simulink model "RadarSimulinkProjectRev008"  (R2024a)
settings: Solver=VariableStepAuto  StartTime=0.0  StopTime=0.0125  RelTol=1e-3
values from neighbouring files (symbols this model uses):
  AngleTime = SweepTime/10    (= 10000)    [InitializationOfVariablesRev000.m]    (also in InitializationOfVariablesRev001.m; InitializationOfVariablesRev002.m = 2000; InitializationOfVariablesRev003.m = 20000; InitializationOfVariablesRev004.m = 2097152)
  ASR_LUT = Rsamp    [InitializationOfVariablesRev003.m]    (also in InitializationOfVariablesRev004.m = round((R*2*SystemFs)/c); InitializationOfVariablesRev005.m = round((R*2*SystemFs)/c))
  Btn_Debounce = 20000    [InitializationOfVariablesRev003.m]    (also in InitializationOfVariablesRev004.m; InitializationOfVariablesRev005.m)
  ChirpNc = 128    [InitializationOfVariablesRev004.m]    (also in InitializationOfVariablesRev005.m)
  ChirpSizeLength = length(FCW)    [InitializationOfVariablesRev004.m]    (also in InitializationOfVariablesRev005.m = 16384)
  DeciFactor = 8    [InitializationOfVariablesRev005.m]
  FCW = [FCW_p1, FCW_p2]    [InitializationOfVariablesRev002.m]    (also in InitializationOfVariablesRev003.m; InitializationOfVariablesRev004.m = interp1(1:length(FCW_base), FCW_base,      linspace(1, lengt; InitializationOfVariablesRev005.m = f / SystemFs)
  filt1divide = sum(h1_int)    [InitializationOfVariablesRev004.m]
  RXFFTLength = 4096    [InitializationOfVariablesRev003.m]    (also in InitializationOfVariablesRev004.m = 1024; InitializationOfVariablesRev005.m = 2048)
  SweepTime = 100000    [InitializationOfVariablesRev000.m]    (also in InitializationOfVariablesRev001.m; InitializationOfVariablesRev002.m = 20000; InitializationOfVariablesRev003.m = 200000; InitializationOfVariablesRev004.m = 23068672)
undefined symbols (not defined in the file or in its folder): SignalGenerationForAnalysis, Subsystem, xc7a200tfbg676
libraries: hdlBasic x362, hdlDSPIP x15, hdlUtilities x11, vmcUtilities x1
(part 3 of 4)

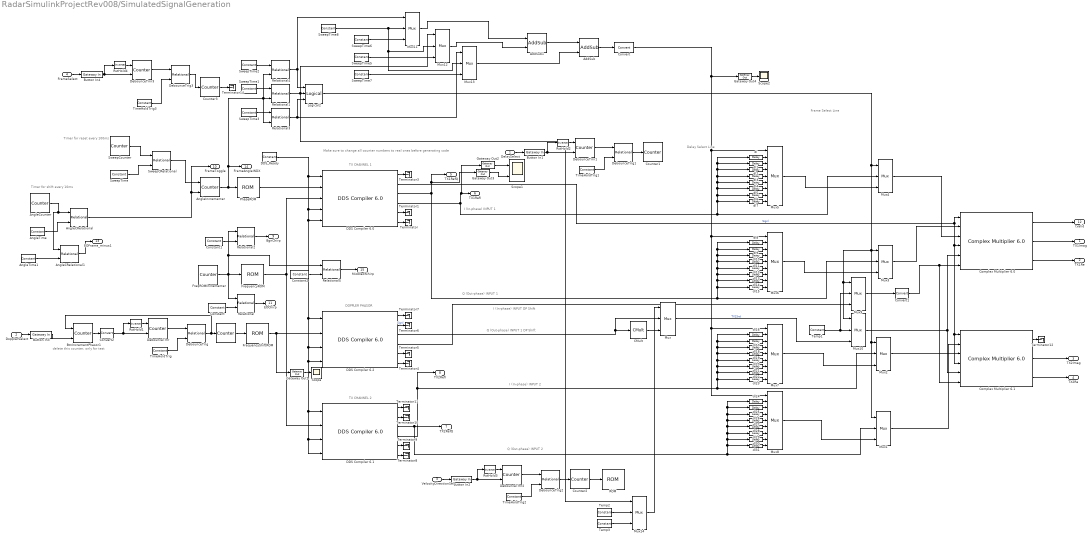
== system RadarSimulinkProjectRev008/SimulatedSignalGeneration ==
  note: delete this counter, only for test
  note: TX CHANNEL 1
  note: Frame Select Line
  note: Make sure to change all counter numbers to real ones before generating code
  note: Timer for shift every 10ms
  note: Timer for reset every 100ms
  note: I (In-phase) INPUT 1
  note: Q (Out-phase) INPUT 1
  note: Q (Out-phase) INPUT 2
  note: Q (Out-phase) INPUT 1 DP Shift
  note: I (In-phase) INPUT DP Shift
  note: I (In-phase) INPUT 2
  note: Delay Select Line
  note: TX CHANNEL 2
  note: DOPPLER PHASOR
  DelaySelect : Inport
  DopplerSelect : Inport  Port=2
  VelocityDirectionSel : Inport  Port=3
  FrameSelect : Inport  Port=4
  " " : hdlBasic/Counter  cnt_type=Count limited  cnt_to=8  operation=Up  start_count=6  cnt_by_val=1  arith_type=Unsigned  n_bits=4  bin_pt=0  load_pin=off  rst=off  en=on  explicit_period=Explicit  period=P1  use_behavioral_HDL=off  implementation=Fabric  XmcBlockStatus=1  maskContainerNames=group1  block_type=counter  block_config=sysgen:Counter_config  block_width=531  block_height=1023
  AddSub : hdlBasic/AddSub  mode=Addition  use_carryin=off  use_carryout=off  en=off  latency=0  precision=Full  arith_type=Unsigned  n_bits=16  bin_pt=14  quantization=Truncate  overflow=Wrap  use_behavioral_HDL=off  hw_selection=Fabric  pipelined=off  XmcBlockStatus=1  maskContainerNames=tabcontainer1  block_type=addsub  block_config=sysgen:Addsub_config
  AddSub1 : hdlBasic/AddSub  mode=Addition  use_carryin=off  use_carryout=off  en=off  latency=0  precision=Full  arith_type=Unsigned  n_bits=16  bin_pt=14  quantization=Truncate  overflow=Wrap  use_behavioral_HDL=off  hw_selection=Fabric  pipelined=off  XmcBlockStatus=1  maskContainerNames=tabcontainer1  block_type=addsub  block_config=sysgen:Addsub_config
  AngleCRelational : hdlBasic/Relational  mode=a=b  op_type=Bool  en=off  latency=0  XmcBlockStatus=1  maskContainerNames=tabcontainer1  block_type=relational  block_config=sysgen:Relational_config
  AngleCRelational1 : hdlBasic/Relational  mode=a=b  op_type=Bool  en=off  latency=0  XmcBlockStatus=1  maskContainerNames=tabcontainer1  block_type=relational  block_config=sysgen:Relational_config
  AngleCounter : hdlBasic/Counter  cnt_type=Count limited  cnt_to=AngleTime-1  operation=Up  start_count=0  cnt_by_val=1  arith_type=Unsigned  n_bits=32  bin_pt=0  load_pin=off  rst=off  en=off  explicit_period=Explicit  period=P1  use_behavioral_HDL=off  implementation=Fabric  XmcBlockStatus=1  maskContainerNames=group1  block_type=counter  block_config=sysgen:Counter_config  block_width=531  block_height=1023
  AngleIncrementer : hdlBasic/Counter  cnt_type=Count limited  cnt_to=10  operation=Up  start_count=0  cnt_by_val=1  arith_type=Unsigned  n_bits=4  bin_pt=0  load_pin=off  rst=on  en=on  explicit_period=Explicit  period=P1  use_behavioral_HDL=off  implementation=Fabric  XmcBlockStatus=1  maskContainerNames=group1  block_type=counter  block_config=sysgen:Counter_config  block_width=531  block_height=1023
  AngleTime : hdlBasic/Constant  const=AngleTime-1  gui_display_data_type=Fixed-point  arith_type=Unsigned  n_bits=24  bin_pt=0  preci_type=Single  exp_width=8  frac_width=24  explicit_period=off  period=1  XmcBlockStatus=1  maskContainerNames=tabcontainer1  block_type=constant  block_config=sysgen:Constant_config
  AngleTime1 : hdlBasic/Constant  const=AngleTime-2  gui_display_data_type=Fixed-point  arith_type=Unsigned  n_bits=24  bin_pt=0  preci_type=Single  exp_width=8  frac_width=24  explicit_period=off  period=1  XmcBlockStatus=1  maskContainerNames=tabcontainer1  block_type=constant  block_config=sysgen:Constant_config
  BtnIncrementPhasor1 : hdlBasic/Counter  cnt_type=Count limited  cnt_to=1  operation=Up  start_count=0  cnt_by_val=1  arith_type=Unsigned  n_bits=1  bin_pt=0  load_pin=off  rst=on  en=on  explicit_period=Explicit  period=P1  use_behavioral_HDL=off  implementation=Fabric  XmcBlockStatus=1  maskContainerNames=group1  block_type=counter  block_config=sysgen:Counter_config  block_width=531  block_height=1023
  Button In{1..4} (4 alike) : hdlBasic/Gateway In  gui_display_data_type=Boolean  arith_type=Boolean  n_bits=16  bin_pt=14  preci_type=Single  exp_width=8  frac_width=24  rows=1  columns=1  quantization="Round  (unbiased: +/- Inf)"  overflow=Saturate  period=P1  UseAsADC=off  ADCChannel='1'  interface=None  automatic_assignment=on  address_offset=hex2dec('00')  intf_name=''  intf_description=''  default_value=0  timing_constraint=None  locs_specified=off  LOCs={}  io_standard={}  inherit_from_input=off  hdl_port=on  XmcBlockStatus=1  maskContainerNames=group4  block_type=gatewayin  block_config=sysgen:gateway_in_config  block_width_w=590  block_height_w=620  block_width=640  block_height=850
  CMult : hdlBasic/CMult  const=-1  gui_display_data_type=Fixed-point  const_n_bits=1  const_bin_pt=0  float_type=Single  exp_bits=8  fraction_bits=24  en=off  latency=0  precision=Full  arith_type="Signed  (2's comp)"  n_bits=16  bin_pt=14  quantization=Truncate  overflow=Wrap  use_behavioral_HDL=off  mem_type=Distributed RAM  pipeline=off  XmcBlockStatus=1  maskContainerNames=tabcontainer1  block_type=cmult  block_config=sysgen:CMult_config
      settings: infoedit=[]
  Complex Multiplier 6.0 : hdlDSPIP/Complex Multiplier 6.0   datatype=integer  hasatlast=off  hasatuser=off  atuserwidth=1  hasbtlast=off  hasbtuser=off  btuserwidth=1  multtype=Use_Mults  optimizegoal=Resources  flowcontrol=NonBlocking  outputwidth=34  roundmode=Truncate  hasctrltlast=off  hasctrltuser=off  ctrltuserwidth=1  outtlastbehv=Null  latencyconfig=Manual  minimumlatency=50  aclken=off  aresetn=off  trim_axipin_name=on  simulation_type=hybrid_sim  simulation_model=sysgen:cmpy_v6_0  data_path_portlist={ 's_axis_a_tdata_real', 's_axis_a_tdata_imag', 's_axis_b_tdata_real', 's_axis_b_tdata_imag', 's_axis_ctrl_tdata_rounding_bit', 'm_axis_dout_tdata_real', 'm_axis_dout_tdata_imag' }  aportwidth=63  bportwidth=63  ip_name=Complex Multiplier  ip_version=6.0  dsptool_ready=true  ipcore_usecache=true  ipcore_useipmodelcache=true  ipcore_verbose=false  ipcore_latency_parameter='minimumlatency'  wrapper_available=true  port_translation_map={ 'aclken' => 'en', 'aresetn' => 'rst'}  XmcBlockStatus=1  maskContainerNames=tabcontainer1  block_type=cmpy_v6_0  block_config=sysgen:rodinimport_config
  Complex Multiplier 6.1 : hdlDSPIP/Complex Multiplier 6.0   datatype=integer  hasatlast=off  hasatuser=off  atuserwidth=1  hasbtlast=off  hasbtuser=off  btuserwidth=1  multtype=Use_Mults  optimizegoal=Resources  flowcontrol=NonBlocking  outputwidth=34  roundmode=Truncate  hasctrltlast=off  hasctrltuser=off  ctrltuserwidth=1  outtlastbehv=Null  latencyconfig=Manual  minimumlatency=50  aclken=off  aresetn=off  trim_axipin_name=on  simulation_type=hybrid_sim  simulation_model=sysgen:cmpy_v6_0  data_path_portlist={ 's_axis_a_tdata_real', 's_axis_a_tdata_imag', 's_axis_b_tdata_real', 's_axis_b_tdata_imag', 's_axis_ctrl_tdata_rounding_bit', 'm_axis_dout_tdata_real', 'm_axis_dout_tdata_imag' }  aportwidth=63  bportwidth=63  ip_name=Complex Multiplier  ip_version=6.0  dsptool_ready=true  ipcore_usecache=true  ipcore_useipmodelcache=true  ipcore_verbose=false  ipcore_latency_parameter='minimumlatency'  wrapper_available=true  port_translation_map={ 'aclken' => 'en', 'aresetn' => 'rst'}  XmcBlockStatus=1  maskContainerNames=tabcontainer1  block_type=cmpy_v6_0  block_config=sysgen:rodinimport_config
  Constant : hdlBasic/Constant  const=length(FCW)-1  gui_display_data_type=Fixed-point  arith_type=Unsigned  n_bits=14  bin_pt=0  preci_type=Single  exp_width=8  frac_width=24  explicit_period=off  period=1  XmcBlockStatus=1  maskContainerNames=tabcontainer1  block_type=constant  block_config=sysgen:Constant_config
  Constant1 : hdlBasic/Constant  const=0  gui_display_data_type=Fixed-point  arith_type=Unsigned  n_bits=12  bin_pt=0  preci_type=Single  exp_width=8  frac_width=24  explicit_period=off  period=1  XmcBlockStatus=1  maskContainerNames=tabcontainer1  block_type=constant  block_config=sysgen:Constant_config
  Constant2 : hdlBasic/Constant  const=(length(FCW)/2)-1  gui_display_data_type=Fixed-point  arith_type=Unsigned  n_bits=13  bin_pt=0  preci_type=Single  exp_width=8  frac_width=24  explicit_period=off  period=1  XmcBlockStatus=1  maskContainerNames=tabcontainer1  block_type=constant  block_config=sysgen:Constant_config
  Convert : hdlBasic/Convert  gui_display_data_type=Fixed-point  arith_type=Unsigned  n_bits=3  bin_pt=0  float_type=Single  exp_bits=8  fraction_bits=24  quantization=Truncate  overflow=Wrap  en=off  latency=0  pipeline=off  XmcBlockStatus=1  maskContainerNames=group2  block_type=convert  block_config=sysgen:Convert_config  block_width=595  block_height=885
  Convert1 : hdlBasic/Convert  gui_display_data_type=Fixed-point  arith_type=Signed (2's comp)  n_bits=17  bin_pt=15  float_type=Single  exp_bits=8  fraction_bits=24  quantization=Truncate  overflow=Saturate  en=off  latency=0  pipeline=off  XmcBlockStatus=1  maskContainerNames=group2  block_type=convert  block_config=sysgen:Convert_config  block_width=595  block_height=885
  Convert2 : hdlBasic/Convert  gui_display_data_type=Boolean  arith_type=Boolean  n_bits=17  bin_pt=15  float_type=Single  exp_bits=8  fraction_bits=24  quantization=Truncate  overflow=Wrap  en=off  latency=0  pipeline=off  XmcBlockStatus=1  maskContainerNames=group2  block_type=convert  block_config=sysgen:Convert_config  block_width=595  block_height=885
  Counter1 : hdlBasic/Counter  cnt_type=Count limited  cnt_to=7  operation=Up  start_count=0  cnt_by_val=1  arith_type=Unsigned  n_bits=3  bin_pt=0  load_pin=off  rst=off  en=on  explicit_period=Explicit  period=P1  use_behavioral_HDL=off  implementation=Fabric  XmcBlockStatus=1  maskContainerNames=group1  block_type=counter  block_config=sysgen:Counter_config  block_width=531  block_height=1023
  Counter2 : hdlBasic/Counter  cnt_type=Count limited  cnt_to=1  operation=Up  start_count=0  cnt_by_val=1  arith_type=Unsigned  n_bits=1  bin_pt=0  load_pin=off  rst=off  en=on  explicit_period=Explicit  period=P1  use_behavioral_HDL=off  implementation=Fabric  XmcBlockStatus=1  maskContainerNames=group1  block_type=counter  block_config=sysgen:Counter_config  block_width=531  block_height=1023
  Counter3 : hdlBasic/Counter  cnt_type=Count limited  cnt_to=10  operation=Up  start_count=0  cnt_by_val=1  arith_type=Unsigned  n_bits=4  bin_pt=0  load_pin=off  rst=off  en=on  explicit_period=Explicit  period=P1  use_behavioral_HDL=off  implementation=Fabric  XmcBlockStatus=1  maskContainerNames=group1  block_type=counter  block_config=sysgen:Counter_config  block_width=531  block_height=1023
  DDS Compiler 6.0 : hdlDSPIP/DDS Compiler 6.0   partspresent=Phase_Generator_and_SIN_COS_LUT  dds_clock_rate=200  channels=1  mode_of_operation=Standard  output_type=Integer  modulus=9  parameter_entry=Hardware_Parameters  spurious_free_dynamic_range=45  frequency_resolution=0.4  noise_shaping=None  phase_width=24  output_width=16  output_selection=Sine_and_Cosine  negative_sine=off  negative_cosine=off  amplitude_mode=Full_Range  memory_type=Auto  optimization_goal=Auto  dsp48_use=Minimal  resync=off  latency_configuration=Auto  latency=1  has_phase_out=on  has_aclken=off  has_aresetn=off  explicit_period=on  period=P1  data_has_tlast=Not_Required  has_tready=on  s_phase_has_tuser=Not_Required  m_data_has_tuser=Not_Required  m_phase_has_tuser=Not_Required  s_phase_tuser_width=1  output_form=Twos_Complement  s_config_sync_mode=On_Vector  phase_increment=Streaming  output_frequency1=0  output_frequency2=0  output_frequency3=0  output_frequency4=0  output_frequency5=0  output_frequency6=0  output_frequency7=0  output_frequency8=0  output_frequency9=0  output_frequency10=0  output_frequency11=0  output_frequency12=0  output_frequency13=0  output_frequency14=0  output_frequency15=0  output_frequency16=0  pinc1='0'  pinc2='0'  pinc3='0'  pinc4='0'  pinc5='0'  pinc6='0'  pinc7='0'  pinc8='0'  pinc9='0'  pinc10='0'  pinc11='0'  pinc12='0'  pinc13='0'  pinc14='0'  pinc15='0'  pinc16='0'  phase_offset=Streaming  phase_offset_angles1=0  phase_offset_angles2=0  phase_offset_angles3=0  phase_offset_angles4=0  phase_offset_angles5=0  phase_offset_angles6=0  phase_offset_angles7=0  phase_offset_angles8=0  phase_offset_angles9=0  phase_offset_angles10=0  phase_offset_angles11=0  phase_offset_angles12=0  phase_offset_angles13=0  phase_offset_angles14=0  phase_offset_angles15=0  phase_offset_angles16=0  poff1='0'  poff2='0'  poff3='0'  poff4='0'  poff5='0'  poff6='0'  poff7='0'  poff8='0'  poff9='0'  poff10='0'  poff11='0'  poff12='0'  poff13='0'  poff14='0'  poff15='0'  poff16='0'  trim_axipin_name=on  simulation_type=hybrid_sim  simulation_model=sysgen:xddsv6_0_cmodel  data_path_portlist={ 's_axis_config_tdata_poff', 's_axis_config_tdata_chan0_poff', 's_axis_config_tdata_pinc', 's_axis_config_tdata_chan0_pinc', 's_axis_phase_tdata_resync', 's_axis_phase_tdata_chan0_resync', 's_axis_phase_tdata_poff', 's_axis_phase_tdata_chan0_poff', 's_axis_phase_tdata_pinc', 's_axis_phase_tdata_chan0_pinc', 's_axis_phase_tdata_phase_in', 'm_axis_data_tdata_sine', 'm_axis_data_tdata_chan0_sine', 'm_axis_data_tdata_cosine', 'm_axis_data_tdata_chan0_cosine', 'm_axis_phase_tdata_phase_out', 'm_axis_phase_tdata_chan0_phase_out'}  por_mode=false  gui_behaviour=Sysgen  ip_name=DDS Compiler  ip_version=6.0  dsptool_ready=true  wrapper_available=true  port_translation_map={ 'aclken' => 'en', 'aresetn' => 'rst' }  ipcore_usecache=true  ipcore_useipmodelcache=true  ipcore_xco_need_fpga_part=true  ipcore_fpga_part=[]  ipcore_verbose=false  XmcBlockStatus=1  maskContainerNames=tabcontainer1  block_type=dds_compiler_v6_0  block_config=sysgen:rodinimport_config  block_width=760
  DDS Compiler 6.1 : hdlDSPIP/DDS Compiler 6.0   partspresent=Phase_Generator_and_SIN_COS_LUT  dds_clock_rate=200  channels=1  mode_of_operation=Standard  output_type=Integer  modulus=9  parameter_entry=Hardware_Parameters  spurious_free_dynamic_range=45  frequency_resolution=0.4  noise_shaping=None  phase_width=24  output_width=16  output_selection=Sine_and_Cosine  negative_sine=off  negative_cosine=off  amplitude_mode=Full_Range  memory_type=Auto  optimization_goal=Auto  dsp48_use=Minimal  resync=off  latency_configuration=Auto  latency=1  has_phase_out=on  has_aclken=off  has_aresetn=off  explicit_period=on  period=P1  data_has_tlast=Not_Required  has_tready=on  s_phase_has_tuser=Not_Required  m_data_has_tuser=Not_Required  m_phase_has_tuser=Not_Required  s_phase_tuser_width=1  output_form=Twos_Complement  s_config_sync_mode=On_Vector  phase_increment=Streaming  output_frequency1=0  output_frequency2=0  output_frequency3=0  output_frequency4=0  output_frequency5=0  output_frequency6=0  output_frequency7=0  output_frequency8=0  output_frequency9=0  output_frequency10=0  output_frequency11=0  output_frequency12=0  output_frequency13=0  output_frequency14=0  output_frequency15=0  output_frequency16=0  pinc1='0'  pinc2='0'  pinc3='0'  pinc4='0'  pinc5='0'  pinc6='0'  pinc7='0'  pinc8='0'  pinc9='0'  pinc10='0'  pinc11='0'  pinc12='0'  pinc13='0'  pinc14='0'  pinc15='0'  pinc16='0'  phase_offset=Fixed  phase_offset_angles1=0  phase_offset_angles2=0  phase_offset_angles3=0  phase_offset_angles4=0  phase_offset_angles5=0  phase_offset_angles6=0  phase_offset_angles7=0  phase_offset_angles8=0  phase_offset_angles9=0  phase_offset_angles10=0  phase_offset_angles11=0  phase_offset_angles12=0  phase_offset_angles13=0  phase_offset_angles14=0  phase_offset_angles15=0  phase_offset_angles16=0  poff1='0'  poff2='0'  poff3='0'  poff4='0'  poff5='0'  poff6='0'  poff7='0'  poff8='0'  poff9='0'  poff10='0'  poff11='0'  poff12='0'  poff13='0'  poff14='0'  poff15='0'  poff16='0'  trim_axipin_name=on  simulation_type=hybrid_sim  simulation_model=sysgen:xddsv6_0_cmodel  data_path_portlist={ 's_axis_config_tdata_poff', 's_axis_config_tdata_chan0_poff', 's_axis_config_tdata_pinc', 's_axis_config_tdata_chan0_pinc', 's_axis_phase_tdata_resync', 's_axis_phase_tdata_chan0_resync', 's_axis_phase_tdata_poff', 's_axis_phase_tdata_chan0_poff', 's_axis_phase_tdata_pinc', 's_axis_phase_tdata_chan0_pinc', 's_axis_phase_tdata_phase_in', 'm_axis_data_tdata_sine', 'm_axis_data_tdata_chan0_sine', 'm_axis_data_tdata_cosine', 'm_axis_data_tdata_chan0_cosine', 'm_axis_phase_tdata_phase_out', 'm_axis_phase_tdata_chan0_phase_out'}  por_mode=false  gui_behaviour=Sysgen  ip_name=DDS Compiler  ip_version=6.0  dsptool_ready=true  wrapper_available=true  port_translation_map={ 'aclken' => 'en', 'aresetn' => 'rst' }  ipcore_usecache=true  ipcore_useipmodelcache=true  ipcore_xco_need_fpga_part=true  ipcore_fpga_part=[]  ipcore_verbose=false  XmcBlockStatus=1  maskContainerNames=tabcontainer1  block_type=dds_compiler_v6_0  block_config=sysgen:rodinimport_config  block_width=760
  DDS Compiler 6.2 : hdlDSPIP/DDS Compiler 6.0   partspresent=Phase_Generator_and_SIN_COS_LUT  dds_clock_rate=200  channels=1  mode_of_operation=Standard  output_type=Integer  modulus=9  parameter_entry=Hardware_Parameters  spurious_free_dynamic_range=45  frequency_resolution=0.4  noise_shaping=None  phase_width=24  output_width=16  output_selection=Sine_and_Cosine  negative_sine=off  negative_cosine=off  amplitude_mode=Full_Range  memory_type=Auto  optimization_goal=Auto  dsp48_use=Minimal  resync=off  latency_configuration=Auto  latency=1  has_phase_out=on  has_aclken=off  has_aresetn=off  explicit_period=on  period=P1  data_has_tlast=Not_Required  has_tready=on  s_phase_has_tuser=Not_Required  m_data_has_tuser=Not_Required  m_phase_has_tuser=Not_Required  s_phase_tuser_width=1  output_form=Twos_Complement  s_config_sync_mode=On_Vector  phase_increment=Streaming  output_frequency1=0  output_frequency2=0  output_frequency3=0  output_frequency4=0  output_frequency5=0  output_frequency6=0  output_frequency7=0  output_frequency8=0  output_frequency9=0  output_frequency10=0  output_frequency11=0  output_frequency12=0  output_frequency13=0  output_frequency14=0  output_frequency15=0  output_frequency16=0  pinc1='0'  pinc2='0'  pinc3='0'  pinc4='0'  pinc5='0'  pinc6='0'  pinc7='0'  pinc8='0'  pinc9='0'  pinc10='0'  pinc11='0'  pinc12='0'  pinc13='0'  pinc14='0'  pinc15='0'  pinc16='0'  phase_offset=None  phase_offset_angles1=0  phase_offset_angles2=0  phase_offset_angles3=0  phase_offset_angles4=0  phase_offset_angles5=0  phase_offset_angles6=0  phase_offset_angles7=0  phase_offset_angles8=0  phase_offset_angles9=0  phase_offset_angles10=0  phase_offset_angles11=0  phase_offset_angles12=0  phase_offset_angles13=0  phase_offset_angles14=0  phase_offset_angles15=0  phase_offset_angles16=0  poff1='0'  poff2='0'  poff3='0'  poff4='0'  poff5='0'  poff6='0'  poff7='0'  poff8='0'  poff9='0'  poff10='0'  poff11='0'  poff12='0'  poff13='0'  poff14='0'  poff15='0'  poff16='0'  trim_axipin_name=on  simulation_type=hybrid_sim  simulation_model=sysgen:xddsv6_0_cmodel  data_path_portlist={ 's_axis_config_tdata_poff', 's_axis_config_tdata_chan0_poff', 's_axis_config_tdata_pinc', 's_axis_config_tdata_chan0_pinc', 's_axis_phase_tdata_resync', 's_axis_phase_tdata_chan0_resync', 's_axis_phase_tdata_poff', 's_axis_phase_tdata_chan0_poff', 's_axis_phase_tdata_pinc', 's_axis_phase_tdata_chan0_pinc', 's_axis_phase_tdata_phase_in', 'm_axis_data_tdata_sine', 'm_axis_data_tdata_chan0_sine', 'm_axis_data_tdata_cosine', 'm_axis_data_tdata_chan0_cosine', 'm_axis_phase_tdata_phase_out', 'm_axis_phase_tdata_chan0_phase_out'}  por_mode=false  gui_behaviour=Sysgen  ip_name=DDS Compiler  ip_version=6.0  dsptool_ready=true  wrapper_available=true  port_translation_map={ 'aclken' => 'en', 'aresetn' => 'rst' }  ipcore_usecache=true  ipcore_useipmodelcache=true  ipcore_xco_need_fpga_part=true  ipcore_fpga_part=[]  ipcore_verbose=false  XmcBlockStatus=1  maskContainerNames=tabcontainer1  block_type=dds_compiler_v6_0  block_config=sysgen:rodinimport_config  block_width=760
  DDS_Ready : hdlBasic/Constant  const=1  gui_display_data_type=Boolean  arith_type=Boolean  n_bits=24  bin_pt=0  preci_type=Single  exp_width=8  frac_width=24  explicit_period=on  period=P1  XmcBlockStatus=1  maskContainerNames=tabcontainer1  block_type=constant  block_config=sysgen:Constant_config
  DebounceTmr{,1..3} (4 alike) : hdlBasic/Counter  cnt_type=Count limited  cnt_to=Btn_Debounce-1  operation=Up  start_count=0  cnt_by_val=1  arith_type=Unsigned  n_bits=18  bin_pt=0  load_pin=off  rst=on  en=on  explicit_period=Explicit  period=P1  use_behavioral_HDL=off  implementation=Fabric  XmcBlockStatus=1  maskContainerNames=group1  block_type=counter  block_config=sysgen:Counter_config  block_width=531  block_height=1023
  DebounceTrig{,1..3} (4 alike) : hdlBasic/Relational  mode=a=b  op_type=Bool  en=off  latency=1  XmcBlockStatus=1  maskContainerNames=tabcontainer1  block_type=relational  block_config=sysgen:Relational_config
  FreqROMIncrementer : hdlBasic/Counter  cnt_type=Count limited  cnt_to=length(FCW)-1  operation=Up  start_count=0  cnt_by_val=1  arith_type=Unsigned  n_bits=14  bin_pt=0  load_pin=off  rst=off  en=off  explicit_period=Explicit  period=P1  use_behavioral_HDL=off  implementation=Fabric  XmcBlockStatus=1  maskContainerNames=group1  block_type=counter  block_config=sysgen:Counter_config  block_width=531  block_height=1023
  FrequencyROM : hdlBasic/ROM  depth=length(FCW)  initVector=FCW  distributed_mem=Block RAM  rst=off  init_reg=0  en=off  latency=1  gui_display_data_type=Fixed-point  arith_type=Unsigned  n_bits=24  bin_pt=24  preci_type=Double  exp_width=8  frac_width=24  optimize=Area  use_rpm=on  simulation_type=fast_sim  XmcBlockStatus=1  maskContainerNames=tabcontainer1  block_type=sprom  block_config=sysgen:SPROM_config
  FrequencyShiftROM : hdlBasic/ROM  depth=9  initVector=DPShift  distributed_mem=Block RAM  rst=off  init_reg=0  en=off  latency=1  gui_display_data_type=Fixed-point  arith_type=Unsigned  n_bits=24  bin_pt=24  preci_type=Double  exp_width=8  frac_width=24  optimize=Area  use_rpm=on  simulation_type=fast_sim  XmcBlockStatus=1  maskContainerNames=tabcontainer1  block_type=sprom  block_config=sysgen:SPROM_config
  Gateway Out{1..4} (4 alike) : hdlBasic/Gateway Out  inherit_from_input=off  bool_to_boolean=off  hdl_port=on  rows=1  columns=1  UseAsDAC=off  DACChannel='1'  interface=None  automatic_assignment=on  address_offset=hex2dec('00')  intf_name=''  intf_description=''  timing_constraint=None  locs_specified=off  LOCs={}  io_standard={}  XmcBlockStatus=1  maskContainerNames=group4  block_type=gatewayout  block_config=sysgen:gateway_out_config  block_width_w=590  block_height_w=620  block_width=620  block_height=750
  Logical2 : hdlBasic/Logical  logical_function=OR  inputs=3  en=off  latency=0  precision=Full  arith_type=Unsigned  n_bits=16  bin_pt=0  align_bp=on  overflow=[]  quantization=[]  XmcBlockStatus=1  maskContainerNames=tabcontainer1  block_type=logical  block_config=sysgen:Logical_config
  Mux{,1..4,9..14} (11 alike) : hdlBasic/Mux  inputs=2  en=off  latency=0  precision=Full  arith_type=Unsigned  n_bits=16  bin_pt=14  quantization=Truncate  overflow=Wrap  XmcBlockStatus=1  maskContainerNames=tabcontainer1  block_type=mux  block_config=sysgen:Mux_config
  Mux{5..8} (4 alike) : hdlBasic/Mux  inputs=8  en=off  latency=0  precision=Full  arith_type=Unsigned  n_bits=16  bin_pt=14  quantization=Truncate  overflow=Wrap  XmcBlockStatus=1  maskContainerNames=tabcontainer1  block_type=mux  block_config=sysgen:Mux_config
  PhaseROM : hdlBasic/ROM  depth=11  initVector=phi_norm  distributed_mem=Block RAM  rst=off  init_reg=0  en=off  latency=1  gui_display_data_type=Fixed-point  arith_type=Unsigned  n_bits=24  bin_pt=24  preci_type=Double  exp_width=8  frac_width=24  optimize=Area  use_rpm=on  simulation_type=fast_sim  XmcBlockStatus=1  maskContainerNames=tabcontainer1  block_type=sprom  block_config=sysgen:SPROM_config
  ROM : hdlBasic/ROM  depth=2  initVector=[0,1]  distributed_mem=Block RAM  rst=off  init_reg=0  en=off  latency=1  gui_display_data_type=Boolean  arith_type=Boolean  n_bits=16  bin_pt=14  preci_type=Single  exp_width=8  frac_width=24  optimize=Area  use_rpm=on  simulation_type=fast_sim  XmcBlockStatus=1  maskContainerNames=tabcontainer1  block_type=sprom  block_config=sysgen:SPROM_config
  Relational : hdlBasic/Relational  mode=a=b  op_type=Bool  en=off  latency=0  XmcBlockStatus=1  maskContainerNames=tabcontainer1  block_type=relational  block_config=sysgen:Relational_config
  Relational1 : hdlBasic/Relational  mode=a=b  op_type=Bool  en=off  latency=1  XmcBlockStatus=1  maskContainerNames=tabcontainer1  block_type=relational  block_config=sysgen:Relational_config
  Relational2 : hdlBasic/Relational  mode=a=b  op_type=Bool  en=off  latency=0  XmcBlockStatus=1  maskContainerNames=tabcontainer1  block_type=relational  block_config=sysgen:Relational_config
  Relational3 : hdlBasic/Relational  mode=a=b  op_type=Bool  en=off  latency=1  XmcBlockStatus=1  maskContainerNames=tabcontainer1  block_type=relational  block_config=sysgen:Relational_config
  Relational4 : hdlBasic/Relational  mode=a=b  op_type=Bool  en=off  latency=1  XmcBlockStatus=1  maskContainerNames=tabcontainer1  block_type=relational  block_config=sysgen:Relational_config
  Relational5 : hdlBasic/Relational  mode=a=b  op_type=Bool  en=off  latency=0  XmcBlockStatus=1  maskContainerNames=tabcontainer1  block_type=relational  block_config=sysgen:Relational_config
  RstHold{1..4} (4 alike) : hdlBasic/Inverter  en=off  latency=0  XmcBlockStatus=1  maskContainerNames=group2  block_type=inv  block_config=sysgen:Inverter_config
  Scope : Scope
  Scope1 : Scope  NumInputPorts=2
  Scope2 : Scope
  SweepCRelational : hdlBasic/Relational  mode=a=b  op_type=Bool  en=off  latency=0  XmcBlockStatus=1  maskContainerNames=tabcontainer1  block_type=relational  block_config=sysgen:Relational_config
  SweepCounter : hdlBasic/Counter  cnt_type=Count limited  cnt_to=SweepTime-1  operation=Up  start_count=0  cnt_by_val=1  arith_type=Unsigned  n_bits=32  bin_pt=0  load_pin=off  rst=off  en=off  explicit_period=Explicit  period=P1  use_behavioral_HDL=off  implementation=Fabric  XmcBlockStatus=1  maskContainerNames=group1  block_type=counter  block_config=sysgen:Counter_config  block_width=531  block_height=1023
  SweepTime : hdlBasic/Constant  const=SweepTime-1  gui_display_data_type=Fixed-point  arith_type=Unsigned  n_bits=32  bin_pt=0  preci_type=Single  exp_width=8  frac_width=24  explicit_period=off  period=1  XmcBlockStatus=1  maskContainerNames=tabcontainer1  block_type=constant  block_config=sysgen:Constant_config
  SweepTime1 : hdlBasic/Constant  const=5  gui_display_data_type=Fixed-point  arith_type=Unsigned  n_bits=4  bin_pt=0  preci_type=Single  exp_width=8  frac_width=24  explicit_period=off  period=1  XmcBlockStatus=1  maskContainerNames=tabcontainer1  block_type=constant  block_config=sysgen:Constant_config
  SweepTime2 : hdlBasic/Constant  const=0  gui_display_data_type=Fixed-point  arith_type=Unsigned  n_bits=4  bin_pt=0  preci_type=Single  exp_width=8  frac_width=24  explicit_period=off  period=1  XmcBlockStatus=1  maskContainerNames=tabcontainer1  block_type=constant  block_config=sysgen:Constant_config
  SweepTime3 : hdlBasic/Constant  const=9  gui_display_data_type=Fixed-point  arith_type=Unsigned  n_bits=4  bin_pt=0  preci_type=Single  exp_width=8  frac_width=24  explicit_period=off  period=1  XmcBlockStatus=1  maskContainerNames=tabcontainer1  block_type=constant  block_config=sysgen:Constant_config
  SweepTime5 : hdlBasic/Constant  const=2  gui_display_data_type=Fixed-point  arith_type=Unsigned  n_bits=3  bin_pt=0  preci_type=Single  exp_width=8  frac_width=24  explicit_period=off  period=1  XmcBlockStatus=1  maskContainerNames=tabcontainer1  block_type=constant  block_config=sysgen:Constant_config
  SweepTime6 : hdlBasic/Constant  const=4  gui_display_data_type=Fixed-point  arith_type=Unsigned  n_bits=3  bin_pt=0  preci_type=Single  exp_width=8  frac_width=24  explicit_period=off  period=1  XmcBlockStatus=1  maskContainerNames=tabcontainer1  block_type=constant  block_config=sysgen:Constant_config
  SweepTime7 : hdlBasic/Constant  const=7  gui_display_data_type=Fixed-point  arith_type=Unsigned  n_bits=3  bin_pt=0  preci_type=Single  exp_width=8  frac_width=24  explicit_period=off  period=1  XmcBlockStatus=1  maskContainerNames=tabcontainer1  block_type=constant  block_config=sysgen:Constant_config
  SweepTime8 : hdlBasic/Constant  const=0  gui_display_data_type=Fixed-point  arith_type=Unsigned  n_bits=3  bin_pt=0  preci_type=Single  exp_width=8  frac_width=24  explicit_period=off  period=1  XmcBlockStatus=1  maskContainerNames=tabcontainer1  block_type=constant  block_config=sysgen:Constant_config
  Temp1 : hdlBasic/Constant  const=0  gui_display_data_type=Fixed-point  arith_type=Unsigned  n_bits=16  bin_pt=15  preci_type=Single  exp_width=8  frac_width=24  explicit_period=off  period=1  XmcBlockStatus=1  maskContainerNames=tabcontainer1  block_type=constant  block_config=sysgen:Constant_config
  Temp2 : hdlBasic/Constant  const=0  gui_display_data_type=Fixed-point  arith_type=Unsigned  n_bits=1  bin_pt=0  preci_type=Single  exp_width=8  frac_width=24  explicit_period=off  period=1  XmcBlockStatus=1  maskContainerNames=tabcontainer1  block_type=constant  block_config=sysgen:Constant_config
  Temp3 : hdlBasic/Constant  const=1  gui_display_data_type=Fixed-point  arith_type=Unsigned  n_bits=1  bin_pt=0  preci_type=Single  exp_width=8  frac_width=24  explicit_period=off  period=1  XmcBlockStatus=1  maskContainerNames=tabcontainer1  block_type=constant  block_config=sysgen:Constant_config
  Terminator{,1,3..12,14} (13 alike) : Terminator
  TimeHoldTrig{,1..3} (4 alike) : hdlBasic/Constant  const=Btn_Debounce-1  gui_display_data_type=Fixed-point  arith_type=Unsigned  n_bits=18  bin_pt=0  preci_type=Single  exp_width=8  frac_width=24  explicit_period=off  period=1  XmcBlockStatus=1  maskContainerNames=tabcontainer1  block_type=constant  block_config=sysgen:Constant_config
  dl{,8,16,24} (4 alike) : hdlBasic/Delay  rst=off  en=off  latency=ASR_LUT(1)  reg_retiming=off  XmcBlockStatus=1  maskContainerNames=group1  block_type=delay  block_config=sysgen:Delay_config
  dl{1,9,17,25} (4 alike) : hdlBasic/Delay  rst=off  en=off  latency=ASR_LUT(2)  reg_retiming=off  XmcBlockStatus=1  maskContainerNames=group1  block_type=delay  block_config=sysgen:Delay_config
  dl{2,10,18,26} (4 alike) : hdlBasic/Delay  rst=off  en=off  latency=ASR_LUT(3)  reg_retiming=off  XmcBlockStatus=1  maskContainerNames=group1  block_type=delay  block_config=sysgen:Delay_config
  dl{3,11,19,27} (4 alike) : hdlBasic/Delay  rst=off  en=off  latency=ASR_LUT(4)  reg_retiming=off  XmcBlockStatus=1  maskContainerNames=group1  block_type=delay  block_config=sysgen:Delay_config
  dl{4,12,20,28} (4 alike) : hdlBasic/Delay  rst=off  en=off  latency=ASR_LUT(5)  reg_retiming=off  XmcBlockStatus=1  maskContainerNames=group1  block_type=delay  block_config=sysgen:Delay_config
  dl{5,13,21,29} (4 alike) : hdlBasic/Delay  rst=off  en=off  latency=ASR_LUT(6)  reg_retiming=off  XmcBlockStatus=1  maskContainerNames=group1  block_type=delay  block_config=sysgen:Delay_config
  dl{6,14,22,30} (4 alike) : hdlBasic/Delay  rst=off  en=off  latency=ASR_LUT(7)  reg_retiming=off  XmcBlockStatus=1  maskContainerNames=group1  block_type=delay  block_config=sysgen:Delay_config
  dl{7,15,23,31} (4 alike) : hdlBasic/Delay  rst=off  en=off  latency=ASR_LUT(8)  reg_retiming=off  XmcBlockStatus=1  maskContainerNames=group1  block_type=delay  block_config=sysgen:Delay_config
  TX1Imag : Outport
  TX1Re : Outport  Port=2
  TX2Imag : Outport  Port=3
  TX2Re : Outport  Port=4
  TX1RefQ : Outport  Port=5
  TX1RefI : Outport  Port=6
  TX2RefQ : Outport  Port=7
  TX2RefI : Outport  Port=8
  BgnChirp : Outport  Port=9
  FrameToggle : Outport  Port=10
  EOChirp : Outport  Port=11
  tvalid : Outport  Port=12
  EOFrame_minus1 : Outport  Port=13
  FrameAngleINDX : Outport  Port=14
  MiddleofChirp : Outport  Port=15
  wires:
  VelocityDirectionSel/1 -> Button In2/1
  Button In3/1 -> BtnIncrementPhasor1/2
  DDS Compiler 6.1/3 -> Mux1/2, dl29/1, dl24/1, dl25/1, dl26/1, dl27/1, dl28/1, dl30/1, dl31/1, TX2RefQ/1
  DebounceTrig1/1 -> Counter1/1
  FrequencyROM/1 -> DDS Compiler 6.1/2, DDS Compiler 6.0/3
  CMult/1 -> Mux/3
  DebounceTmr/1 -> DebounceTrig/1
  PhaseROM/1 -> DDS Compiler 6.0/2
  DDS_Ready/1 -> DDS Compiler 6.1/4, DDS Compiler 6.1/3, DDS Compiler 6.1/1, DDS Compiler 6.2/4, DDS Compiler 6.2/3, DDS Compiler 6.2/1, DDS Compiler 6.0/5, DDS Compiler 6.0/4, DDS Compiler 6.0/1
  DebounceTrig/1 -> BtnIncrementPhasor1/1, " "/1
  TimeHoldTrig/1 -> DebounceTrig/2
  SweepCounter/1 -> SweepCRelational/1
  Complex Multiplier 6.1/3 -> TX2Re/1
  AngleCounter/1 -> AngleCRelational/1, AngleCRelational1/1
  TimeHoldTrig1/1 -> DebounceTrig1/2
  AngleIncrementer/1 -> FrameAngleINDX/1, Relational4/2, Relational3/2, Relational1/2, PhaseROM/1
  DopplerSelect/1 -> Button In3/1
  Complex Multiplier 6.1/2 -> TX2Imag/1
  " "/1 -> FrequencyShiftROM/1
  Button In1/1 -> RstHold2/1, DebounceTmr1/2
  SweepTime/1 -> SweepCRelational/2
  RstHold1/1 -> DebounceTmr/1
  AngleTime/1 -> AngleCRelational/2
  SweepCRelational/1 -> AngleIncrementer/1
  DebounceTmr2/1 -> DebounceTrig2/1
  DelaySelect/1 -> Button In1/1
  Mux2/1 -> Complex Multiplier 6.1/3
  FrequencyShiftROM/1 -> Gateway Out1/1, DDS Compiler 6.2/2
  TimeHoldTrig2/1 -> DebounceTrig2/2
  RstHold3/1 -> DebounceTmr2/1
  Counter2/1 -> ROM/1
  DDS Compiler 6.0/6 -> Terminator/1
  Complex Multiplier 6.1/1 -> Terminator12/1
  DebounceTmr1/1 -> DebounceTrig1/1
  DebounceTrig2/1 -> Counter2/1
  Mux14/1 -> Mux/1
  Button In2/1 -> RstHold3/1, DebounceTmr2/2
  RstHold2/1 -> DebounceTmr1/1
  DDS Compiler 6.0/2 -> Complex Multiplier 6.1/4, Complex Multiplier 6.1/1, Complex Multiplier 6.0/4, Complex Multiplier 6.0/1  "Signl"
  DDS Compiler 6.1/1 -> Terminator11/1
  DDS Compiler 6.0/5 -> Terminator1/1
  DDS Compiler 6.1/2 -> Terminator10/1
  DDS Compiler 6.2/1 -> Terminator7/1
  DDS Compiler 6.1/5 -> Terminator9/1
  Complex Multiplier 6.0/1 -> tvalid/1
  DDS Compiler 6.1/6 -> Terminator8/1
  DDS Compiler 6.2/6 -> Terminator4/1
  DDS Compiler 6.0/1 -> Terminator3/1
  DDS Compiler 6.2/2 -> Terminator6/1  "Signl"
  DDS Compiler 6.2/5 -> Terminator5/1
  AngleCRelational/1 -> FrameToggle/1, AngleIncrementer/2
  Constant/1 -> Relational/2
  AddSub/1 -> Convert/1
  Mux1/1 -> Complex Multiplier 6.1/2
  Mux3/1 -> Complex Multiplier 6.0/2
  Mux6/1 -> Mux3/3
  Mux5/1 -> Mux4/3
  TimeHoldTrig3/1 -> DebounceTrig3/2
  DebounceTmr3/1 -> DebounceTrig3/1
  FrameSelect/1 -> Button In4/1
  RstHold4/1 -> DebounceTmr3/1
  Button In4/1 -> RstHold4/1, DebounceTmr3/2
  DebounceTrig3/1 -> Counter3/1
  Counter3/1 -> Terminator14/1
  SweepTime1/1 -> Relational1/1
  dl/1 -> Mux5/2
  dl1/1 -> Mux5/3
  dl2/1 -> Mux5/4
  dl3/1 -> Mux5/5
  dl4/1 -> Mux5/6
  dl5/1 -> Mux5/7
  dl6/1 -> Mux5/8
  dl7/1 -> Mux5/9
  dl15/1 -> Mux6/9
  dl10/1 -> Mux6/4
  dl14/1 -> Mux6/8
  dl13/1 -> Mux6/7
  dl11/1 -> Mux6/5
  dl12/1 -> Mux6/6
  DDS Compiler 6.0/3 -> TX1RefQ/1, Gateway Out3/1, Mux3/2, dl15/1, dl14/1, dl13/1, dl12/1, dl11/1, dl10/1, dl9/1, dl8/1
  dl8/1 -> Mux6/2
  dl9/1 -> Mux6/3
  dl23/1 -> Mux7/9
  dl18/1 -> Mux7/4
  dl22/1 -> Mux7/8
  dl21/1 -> Mux7/7
  dl19/1 -> Mux7/5
  dl20/1 -> Mux7/6
  DDS Compiler 6.1/4 -> TX2RefI/1, Mux2/2, dl23/1, dl22/1, dl21/1, dl20/1, dl19/1, dl18/1, dl17/1, dl16/1
  dl16/1 -> Mux7/2
  dl17/1 -> Mux7/3
  Mux7/1 -> Mux2/3
  dl31/1 -> Mux8/9
  dl26/1 -> Mux8/4
  dl30/1 -> Mux8/8
  dl29/1 -> Mux8/7
  dl27/1 -> Mux8/5
  dl28/1 -> Mux8/6
  dl24/1 -> Mux8/2
  dl25/1 -> Mux8/3
  Mux8/1 -> Mux1/3
  Mux10/1 -> Complex Multiplier 6.1/5, Complex Multiplier 6.0/5
  Complex Multiplier 6.0/2 -> TX1Imag/1
  Complex Multiplier 6.0/3 -> TX1Re/1
  DDS Compiler 6.2/4 -> Mux9/3
  Mux9/1 -> Convert1/1
  Temp1/1 -> Mux10/2, Mux9/2
  Convert1/1 -> Complex Multiplier 6.1/6, Complex Multiplier 6.0/6
  DDS Compiler 6.2/3 -> Mux/2, CMult/1
  Mux/1 -> Mux10/3  "TX1SrcI"
  Logical2/1 -> Mux10/1, Mux9/1, Mux1/1, Mux2/1, Mux3/1, Mux4/1
  Mux4/1 -> Complex Multiplier 6.0/3
  Relational/1 -> EOChirp/1
  Constant1/1 -> Relational2/2
  FreqROMIncrementer/1 -> Relational5/1, Relational2/1, Relational/1, FrequencyROM/1
  Relational2/1 -> BgnChirp/1
  AngleTime1/1 -> AngleCRelational1/2
  AngleCRelational1/1 -> EOFrame_minus1/1
  Relational1/1 -> Mux14/1, Mux12/1, Logical2/2
  SweepTime3/1 -> Relational3/1
  SweepTime2/1 -> Relational4/1
  Relational3/1 -> Mux13/1, Logical2/3
  Relational4/1 -> Logical2/1, Mux11/1
  SweepTime5/1 -> Mux12/3
  SweepTime6/1 -> Mux11/3
  SweepTime7/1 -> Mux13/3
  SweepTime8/1 -> Mux13/2, Mux12/2, Mux11/2
  Mux11/1 -> AddSub1/1
  Mux12/1 -> AddSub1/2
  Mux13/1 -> AddSub/2
  AddSub1/1 -> AddSub/1
  Convert/1 -> Gateway Out4/1, Mux8/1, Mux7/1, Mux6/1, Mux5/1
  Temp2/1 -> Mux14/2
  Temp3/1 -> Mux14/3
  Gateway Out1/1 -> Scope/1
  BtnIncrementPhasor1/1 -> Convert2/1
  Convert2/1 -> RstHold1/1, DebounceTmr/2
  DDS Compiler 6.0/4 -> Mux4/2, dl7/1, dl6/1, dl5/1, dl4/1, dl3/1, dl2/1, dl1/1, dl/1, Gateway Out2/1, TX1RefI/1
  Gateway Out3/1 -> Scope1/2
  Gateway Out2/1 -> Scope1/1
  Gateway Out4/1 -> Scope2/1
  Constant2/1 -> Relational5/2
  Relational5/1 -> MiddleofChirp/1

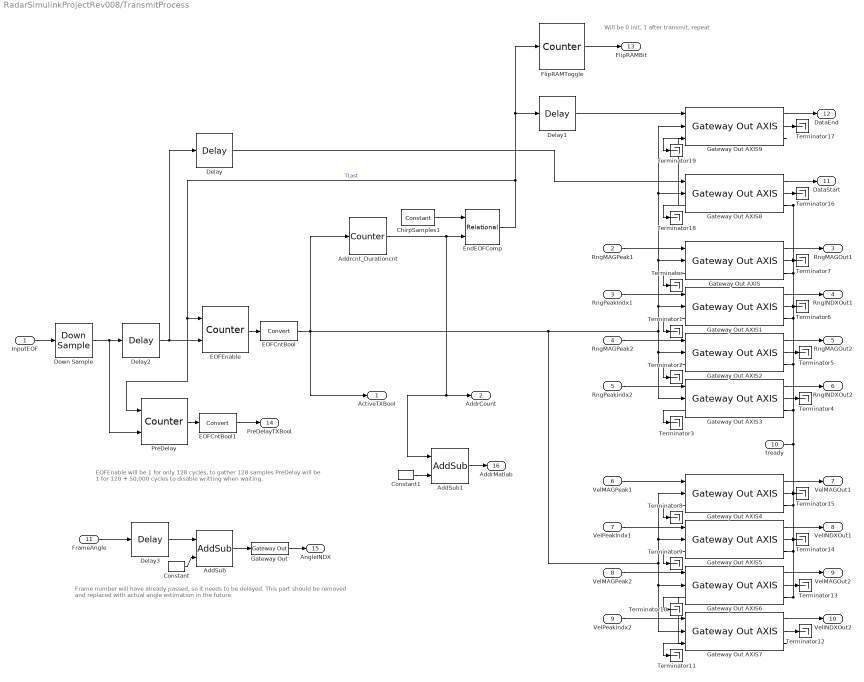
== system RadarSimulinkProjectRev008/TransmitProcess ==
  note: Frame number will have already passed, so it needs to be delayed. This part should be removed and replaced with actual angle estimation in the future.
  note: EOFEnable will be 1 for only 128 cycles, to gather 128 samples
      | PreDelay will be 1 for 128 + 50,000 cycles to disable writting when waiting.
  note: Will be 0 init, 1 after transmit, repeat
  InputEOF : Inport
  RngMAGPeak1 : Inport  Port=2
  RngPeakIndx1 : Inport  Port=3
  RngMAGPeak2 : Inport  Port=4
  RngPeakindx2 : Inport  Port=5
  VelMAGPeak1 : Inport  Port=6
  VelPeakIndx1 : Inport  Port=7
  VelMAGPeak2 : Inport  Port=8
  VelPeakindx2 : Inport  Port=9
  tready : Inport  Port=10
  FrameAngle : Inport  Port=11
  AddSub : hdlBasic/AddSub  mode=Addition  use_carryin=off  use_carryout=off  en=off  latency=1  precision=Full  arith_type=Unsigned  n_bits=16  bin_pt=14  quantization=Truncate  overflow=Wrap  use_behavioral_HDL=off  hw_selection=Fabric  pipelined=off  XmcBlockStatus=1  maskContainerNames=tabcontainer1  block_type=addsub  block_config=sysgen:Addsub_config
  AddSub1 : hdlBasic/AddSub  mode=Addition  use_carryin=off  use_carryout=off  en=off  latency=1  precision=Full  arith_type=Unsigned  n_bits=16  bin_pt=14  quantization=Truncate  overflow=Wrap  use_behavioral_HDL=off  hw_selection=Fabric  pipelined=off  XmcBlockStatus=1  maskContainerNames=tabcontainer1  block_type=addsub  block_config=sysgen:Addsub_config
  Addrcnt_Durationcnt : hdlBasic/Counter  cnt_type=Count limited  cnt_to=ChirpNc-1  operation=Up  start_count=0  cnt_by_val=1  arith_type=Unsigned  n_bits=7  bin_pt=0  load_pin=off  rst=off  en=on  explicit_period=Explicit  period=P2  use_behavioral_HDL=off  implementation=Fabric  XmcBlockStatus=1  maskContainerNames=group1  block_type=counter  block_config=sysgen:Counter_config  block_width=531  block_height=1023
  ChirpSamples1 : hdlBasic/Constant  const=127  gui_display_data_type=Fixed-point  arith_type=Unsigned  n_bits=7  bin_pt=0  preci_type=Single  exp_width=8  frac_width=24  explicit_period=on  period=P2  XmcBlockStatus=1  maskContainerNames=tabcontainer1  block_type=constant  block_config=sysgen:Constant_config
  Constant : hdlBasic/Constant  const=1.0  gui_display_data_type=Fixed-point  arith_type=Unsigned  n_bits=7  bin_pt=0  preci_type=Single  exp_width=8  frac_width=24  explicit_period=off  period=1  XmcBlockStatus=1  maskContainerNames=tabcontainer1  block_type=constant  block_config=sysgen:Constant_config
  Constant1 : hdlBasic/Constant  const=1.0  gui_display_data_type=Fixed-point  arith_type=Unsigned  n_bits=7  bin_pt=0  preci_type=Single  exp_width=8  frac_width=24  explicit_period=off  period=1  XmcBlockStatus=1  maskContainerNames=tabcontainer1  block_type=constant  block_config=sysgen:Constant_config
  Delay : hdlBasic/Delay  rst=off  en=off  latency=1  reg_retiming=off  XmcBlockStatus=1  maskContainerNames=group1  block_type=delay  block_config=sysgen:Delay_config
  Delay1 : hdlBasic/Delay  rst=off  en=off  latency=1  reg_retiming=off  XmcBlockStatus=1  maskContainerNames=group1  block_type=delay  block_config=sysgen:Delay_config
  Delay2 : hdlBasic/Delay  rst=off  en=off  latency=50000  reg_retiming=off  XmcBlockStatus=1  maskContainerNames=group1  block_type=delay  block_config=sysgen:Delay_config
  Delay3 : hdlBasic/Delay  rst=off  en=off  latency=64000  reg_retiming=off  XmcBlockStatus=1  maskContainerNames=group1  block_type=delay  block_config=sysgen:Delay_config
  Down Sample : hdlBasic/Down Sample  sample_ratio=16  sample_phase="Last Value of Frame  (most efficient)"  en=off  rst=off  latency=1  XmcBlockStatus=1  maskContainerNames=group1  block_type=dsamp  block_config=sysgen:Downsample_config
  EOFCntBool : hdlBasic/Convert  gui_display_data_type=Boolean  arith_type=Boolean  n_bits=16  bin_pt=14  float_type=Single  exp_bits=8  fraction_bits=24  quantization=Truncate  overflow=Wrap  en=off  latency=0  pipeline=off  XmcBlockStatus=1  maskContainerNames=group2  block_type=convert  block_config=sysgen:Convert_config  block_width=595  block_height=885
  EOFCntBool1 : hdlBasic/Convert  gui_display_data_type=Boolean  arith_type=Boolean  n_bits=16  bin_pt=14  float_type=Single  exp_bits=8  fraction_bits=24  quantization=Truncate  overflow=Wrap  en=off  latency=0  pipeline=off  XmcBlockStatus=1  maskContainerNames=group2  block_type=convert  block_config=sysgen:Convert_config  block_width=595  block_height=885
  EOFEnable : hdlBasic/Counter  cnt_type=Count limited  cnt_to=1  operation=Up  start_count=0  cnt_by_val=1  arith_type=Unsigned  n_bits=1  bin_pt=0  load_pin=off  rst=on  en=on  explicit_period=Explicit  period=P2  use_behavioral_HDL=off  implementation=Fabric  XmcBlockStatus=1  maskContainerNames=group1  block_type=counter  block_config=sysgen:Counter_config  block_width=531  block_height=1023
  EndEOFComp : hdlBasic/Relational  mode=a=b  op_type=Bool  en=off  latency=0  XmcBlockStatus=1  maskContainerNames=tabcontainer1  block_type=relational  block_config=sysgen:Relational_config
  FlipRAMToggle : hdlBasic/Counter  cnt_type=Count limited  cnt_to=1  operation=Up  start_count=0  cnt_by_val=1  arith_type=Unsigned  n_bits=1  bin_pt=0  load_pin=off  rst=off  en=on  explicit_period=Explicit  period=P2  use_behavioral_HDL=off  implementation=Fabric  XmcBlockStatus=1  maskContainerNames=group1  block_type=counter  block_config=sysgen:Counter_config  block_width=531  block_height=1023
  Gateway Out : hdlBasic/Gateway Out  inherit_from_input=off  bool_to_boolean=off  hdl_port=on  rows=1  columns=1  UseAsDAC=off  DACChannel='1'  interface=None  automatic_assignment=on  address_offset=hex2dec('00')  intf_name=''  intf_description=''  timing_constraint=None  locs_specified=off  LOCs={}  io_standard={}  XmcBlockStatus=1  maskContainerNames=group4  block_type=gatewayout  block_config=sysgen:gateway_out_config  block_width_w=590  block_height_w=620  block_width=620  block_height=750
  Gateway Out AXIS{,1..9} (10 alike) : hdlUtilities/Gateway Out AXIS  mask_sample_period=1  bool_to_boolean=off  block_type=gatewayoutaxi
  PreDelay : hdlBasic/Counter  cnt_type=Count limited  cnt_to=1  operation=Up  start_count=0  cnt_by_val=1  arith_type=Unsigned  n_bits=1  bin_pt=0  load_pin=off  rst=on  en=on  explicit_period=Explicit  period=P2  use_behavioral_HDL=off  implementation=Fabric  XmcBlockStatus=1  maskContainerNames=group1  block_type=counter  block_config=sysgen:Counter_config  block_width=531  block_height=1023
  Terminator{,1..19} (20 alike) : Terminator
  ActiveTXBool : Outport
  AddrCount : Outport  Port=2
  RngMAGOut1 : Outport  Port=3
  RngINDXOut1 : Outport  Port=4
  RngMAGOut2 : Outport  Port=5
  RngINDXOut2 : Outport  Port=6
  VelMAGOut1 : Outport  Port=7
  VelINDXOut1 : Outport  Port=8
  VelMAGOut2 : Outport  Port=9
  VelINDXOut2 : Outport  Port=10
  DataStart : Outport  Port=11
  DataEnd : Outport  Port=12
  FlipRAMBit : Outport  Port=13
  PreDelayTXBool : Outport  Port=14
  AngleINDX : Outport  Port=15
  AddrMatlab : Outport  Port=16
  wires:
  ChirpSamples1/1 -> EndEOFComp/1
  Gateway Out AXIS/1 -> RngMAGOut1/1
  Gateway Out AXIS2/3 -> Terminator2/1
  Gateway Out AXIS3/1 -> RngINDXOut2/1
  InputEOF/1 -> Down Sample/1
  Gateway Out AXIS1/3 -> Terminator1/1
  Gateway Out AXIS1/1 -> RngINDXOut1/1
  Gateway Out AXIS/2 -> Terminator7/1
  EndEOFComp/1 -> FlipRAMToggle/1, Delay1/1, PreDelay/1, EOFEnable/1  "TLast"
  Gateway Out AXIS2/1 -> RngMAGOut2/1
  EOFEnable/1 -> EOFCntBool/1
  RngMAGPeak2/1 -> Gateway Out AXIS2/1
  Gateway Out AXIS2/2 -> Terminator5/1
  RngPeakIndx1/1 -> Gateway Out AXIS1/1
  RngMAGPeak1/1 -> Gateway Out AXIS/1
  Gateway Out AXIS1/2 -> Terminator6/1
  RngPeakindx2/1 -> Gateway Out AXIS3/1
  Gateway Out AXIS3/3 -> Terminator3/1
  Gateway Out AXIS3/2 -> Terminator4/1
  Gateway Out AXIS/3 -> Terminator/1
  Gateway Out AXIS7/3 -> Terminator11/1
  VelPeakindx2/1 -> Gateway Out AXIS7/1
  Gateway Out AXIS6/3 -> Terminator10/1
  VelMAGPeak2/1 -> Gateway Out AXIS6/1
  Gateway Out AXIS5/2 -> Terminator14/1
  Gateway Out AXIS6/1 -> VelMAGOut2/1
  Gateway Out AXIS7/1 -> VelINDXOut2/1
  Gateway Out AXIS5/1 -> VelINDXOut1/1
  EOFCntBool/1 -> Addrcnt_Durationcnt/1, Gateway Out AXIS5/2, Gateway Out AXIS4/2, Gateway Out AXIS7/2, Gateway Out AXIS6/2, Gateway Out AXIS1/2, Gateway Out AXIS9/2, Gateway Out AXIS8/2, Gateway Out AXIS/2, Gateway Out AXIS3/2, Gateway Out AXIS2/2, ActiveTXBool/1
  VelPeakIndx1/1 -> Gateway Out AXIS5/1
  Gateway Out AXIS4/3 -> Terminator8/1
  Gateway Out AXIS6/2 -> Terminator13/1
  VelMAGPeak1/1 -> Gateway Out AXIS4/1
  Gateway Out AXIS7/2 -> Terminator12/1
  Gateway Out AXIS4/1 -> VelMAGOut1/1
  Gateway Out AXIS5/3 -> Terminator9/1
  Gateway Out AXIS4/2 -> Terminator15/1
  tready/1 -> Gateway Out AXIS5/3, Gateway Out AXIS7/3, Gateway Out AXIS6/3, Gateway Out AXIS4/3, Gateway Out AXIS9/3, Gateway Out AXIS8/3, Gateway Out AXIS/3, Gateway Out AXIS1/3, Gateway Out AXIS2/3, Gateway Out AXIS3/3
  Gateway Out AXIS8/1 -> DataStart/1
  Gateway Out AXIS8/2 -> Terminator16/1
  Gateway Out AXIS9/1 -> DataEnd/1
  Gateway Out AXIS9/2 -> Terminator17/1
  Gateway Out AXIS8/3 -> Terminator18/1
  Gateway Out AXIS9/3 -> Terminator19/1
  Delay/1 -> Gateway Out AXIS8/1
  Delay1/1 -> Gateway Out AXIS9/1
  Delay2/1 -> Delay/1, EOFEnable/2
  FlipRAMToggle/1 -> FlipRAMBit/1
  PreDelay/1 -> EOFCntBool1/1
  EOFCntBool1/1 -> PreDelayTXBool/1
  FrameAngle/1 -> Delay3/1
  Delay3/1 -> AddSub/1
  Gateway Out/1 -> AngleINDX/1
  Constant/1 -> AddSub/2
  AddSub/1 -> Gateway Out/1
  Addrcnt_Durationcnt/1 -> AddrCount/1, AddSub1/1, EndEOFComp/2
  AddSub1/1 -> AddrMatlab/1
  Constant1/1 -> AddSub1/2
  Down Sample/1 -> PreDelay/2, Delay2/1
